simulink model "simulinkmodell"  (R2015a)
settings: Solver=ode45  StartTime=0.0  StopTime=10.0  RelTol=1e-3
values from neighbouring files (symbols this model uses):
  K = 0.1744    [DiscKal_backup.m]    (also in Untitled.m; kal_init.m; matlab_1.mat = 0.17436818244; matlab_kalman_backup.mat)
  lambda = 0.0657    [DiscKal_backup.m]    (also in Untitled.m; kal_init.m; matlab_kalman_backup.mat)
  T = 0.1    [DiscKal_backup.m]    (also in Sfunctionshell.m; Untitled.m; kal_init.m = 87.1542; matlab_1.mat = 87.1542392511)
undefined symbols (not defined in the file or in its folder): Kw, w0
settings Model: Creator=magho  LastModifiedBy=magho

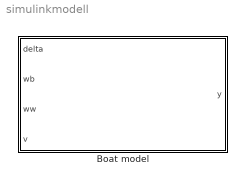
== system simulinkmodell ==
  Boat model : Subsystem

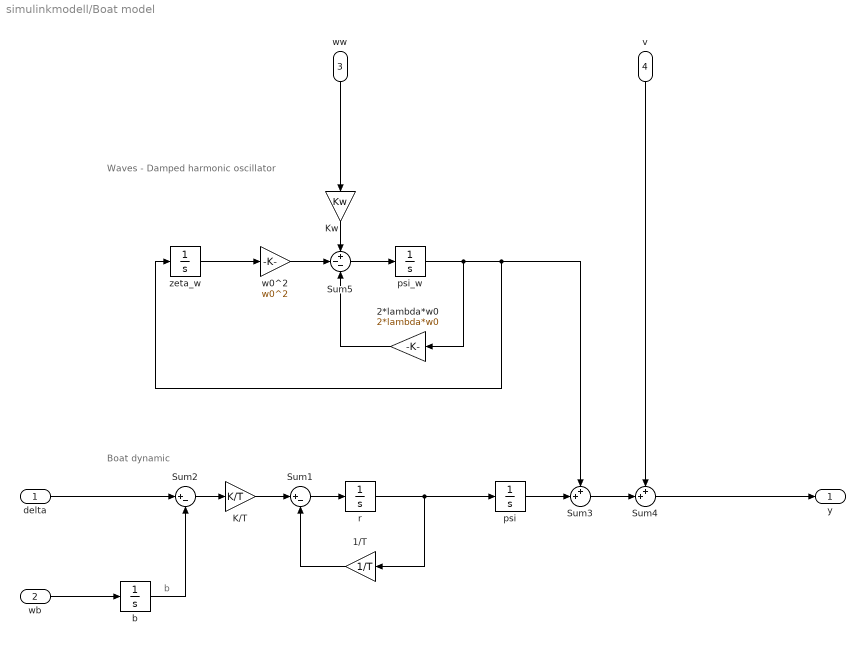
== system simulinkmodell/Boat model ==
  note: Boat dynamic
  note: Waves - Damped harmonic oscillator
  note: b
  delta : Inport
  "wb " : Inport  Port=2
  ww : Inport  Port=3
  v : Inport  Port=4
  1/T : Gain  Gain=1/T
  2*lambda*w0 : Gain  Gain=2*lambda*w0
  K/T : Gain  Gain=K/T
  "Kw " : Gain  Gain=Kw
  Sum1 : Sum  Inputs=|+-
  Sum2 : Sum  Inputs=|+-
  Sum3 : Sum  Inputs=++|
  Sum4 : Sum  Inputs=++|
  Sum5 : Sum  Inputs=+--
  b : Integrator
  psi : Integrator
  psi_w : Integrator
  r : Integrator
  w0^2 : Gain  Gain=w0^2
  zeta_w : Integrator
  y : Outport
  wires:
  psi/1 -> Sum3/2
  Sum3/1 -> Sum4/2
  Sum1/1 -> r/1
  r/1 -> psi/1, 1/T/1
  b/1 -> Sum2/2
  K/T/1 -> Sum1/1
  1/T/1 -> Sum1/2
  Sum4/1 -> y/1
  Sum2/1 -> K/T/1
  "wb "/1 -> b/1
  delta/1 -> Sum2/1
  v/1 -> Sum4/1
  Sum5/1 -> psi_w/1
  psi_w/1 -> zeta_w/1, Sum3/1, 2*lambda*w0/1
  zeta_w/1 -> w0^2/1
  "Kw "/1 -> Sum5/1
  w0^2/1 -> Sum5/2
  2*lambda*w0/1 -> Sum5/3
  ww/1 -> "Kw "/1
